simulink model "EX2"  (R2022b)
settings: Solver=VariableStepAuto  StartTime=0.0  StopTime=10.0  RelTol=1e-3
settings Model: Creator=Dell  LastModifiedBy=Dell

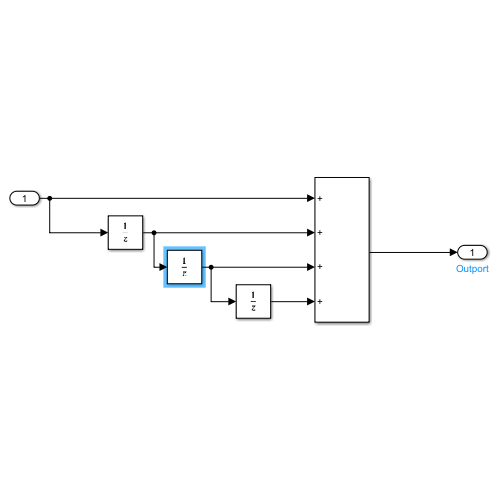
[thumbnail: Simulink's stored preview of the top-level diagram]
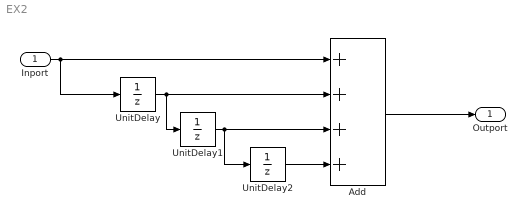
== system EX2 ==
  Inport : Inport
  Add : Sum  Inputs=++++
  UnitDelay : UnitDelay  SampleTime=-1  HasFrameUpgradeWarning=on
  UnitDelay1 : UnitDelay  SampleTime=-1  HasFrameUpgradeWarning=on
  UnitDelay2 : UnitDelay  SampleTime=-1  HasFrameUpgradeWarning=on
  Outport : Outport
  wires:
  Inport/1 -> UnitDelay/1, Add/1
  UnitDelay/1 -> Add/2, UnitDelay1/1
  UnitDelay1/1 -> Add/3, UnitDelay2/1
  UnitDelay2/1 -> Add/4
  Add/1 -> Outport/1
